simulink model "EngDem"  (R2018a)
settings: configuration reference "cs_ert" (kept outside this file)
settings Model: DataDictionary=EngDem.sldd  Creator=zhoutinglin  LastModifiedBy=zhoutinglin

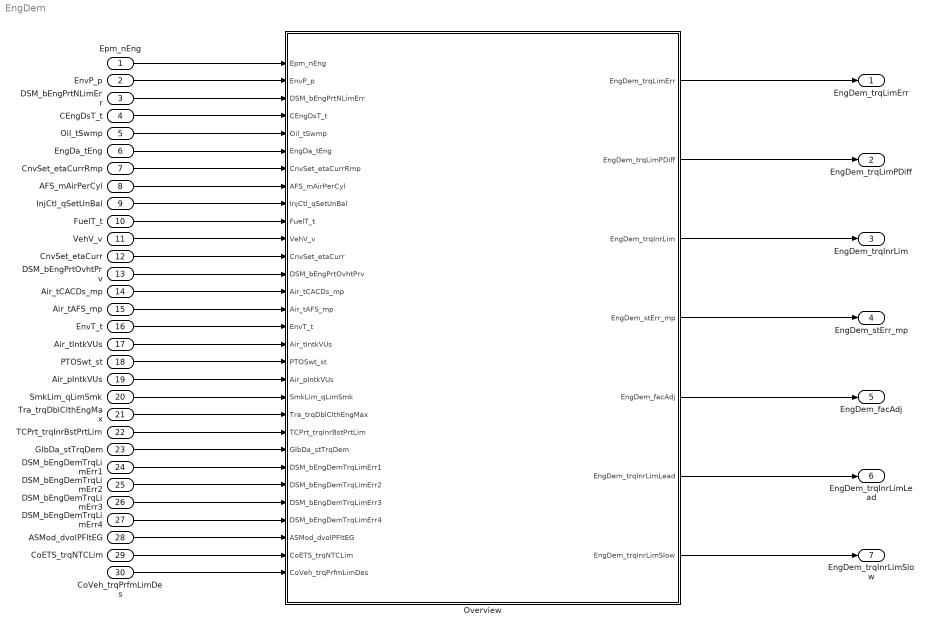
== system EngDem ==
  Epm_nEng : Inport
  EnvP_p : Inport  Port=2
  DSM_bEngPrtNLimErr : Inport  Port=3
  CEngDsT_t : Inport  Port=4
  Oil_tSwmp : Inport  Port=5
  EngDa_tEng : Inport  Port=6
  CnvSet_etaCurrRmp : Inport  Port=7
  AFS_mAirPerCyl : Inport  Port=8
  InjCtl_qSetUnBal : Inport  Port=9
  FuelT_t : Inport  Port=10
  VehV_v : Inport  Port=11
  CnvSet_etaCurr : Inport  Port=12
  DSM_bEngPrtOvhtPrv : Inport  Port=13
  Air_tCACDs_mp : Inport  Port=14
  Air_tAFS_mp : Inport  Port=15
  EnvT_t : Inport  Port=16
  Air_tIntkVUs : Inport  Port=17
  PTOSwt_st : Inport  Port=18
  Air_pIntkVUs : Inport  Port=19
  SmkLim_qLimSmk : Inport  Port=20
  Tra_trqDblClthEngMax : Inport  Port=21
  TCPrt_trqInrBstPrtLim : Inport  Port=22
  GlbDa_stTrqDem : Inport  Port=23
  DSM_bEngDemTrqLimErr1 : Inport  Port=24
  DSM_bEngDemTrqLimErr2 : Inport  Port=25
  DSM_bEngDemTrqLimErr3 : Inport  Port=26
  DSM_bEngDemTrqLimErr4 : Inport  Port=27
  ASMod_dvolPFltEG : Inport  Port=28
  CoETS_trqNTCLim : Inport  Port=29
  CoVeh_trqPrfmLimDes : Inport  Port=30
  Overview : Subsystem
  EngDem_trqLimErr : Outport
  EngDem_trqLimPDiff : Outport  Port=2
  EngDem_trqInrLim : Outport  Port=3
  EngDem_stErr_mp : Outport  Port=4
  EngDem_facAdj : Outport  Port=5
  EngDem_trqInrLimLead : Outport  Port=6
  EngDem_trqInrLimSlow : Outport  Port=7
  wires:
  Epm_nEng/1 -> Overview/1(Epm_nEng)
  EnvP_p/1 -> Overview/2(EnvP_p)
  DSM_bEngPrtNLimErr/1 -> Overview/3(DSM_bEngPrtNLimErr)
  CEngDsT_t/1 -> Overview/4(CEngDsT_t)
  Oil_tSwmp/1 -> Overview/5(Oil_tSwmp)
  EngDa_tEng/1 -> Overview/6(EngDa_tEng)
  CnvSet_etaCurrRmp/1 -> Overview/7(CnvSet_etaCurrRmp)
  AFS_mAirPerCyl/1 -> Overview/8(AFS_mAirPerCyl)
  InjCtl_qSetUnBal/1 -> Overview/9(InjCtl_qSetUnBal)
  FuelT_t/1 -> Overview/10(FuelT_t)
  VehV_v/1 -> Overview/11(VehV_v)
  CnvSet_etaCurr/1 -> Overview/12(CnvSet_etaCurr)
  DSM_bEngPrtOvhtPrv/1 -> Overview/13(DSM_bEngPrtOvhtPrv)
  Air_tCACDs_mp/1 -> Overview/14(Air_tCACDs_mp)
  Air_tAFS_mp/1 -> Overview/15(Air_tAFS_mp)
  EnvT_t/1 -> Overview/16(EnvT_t)
  Air_tIntkVUs/1 -> Overview/17(Air_tIntkVUs)
  PTOSwt_st/1 -> Overview/18(PTOSwt_st)
  Air_pIntkVUs/1 -> Overview/19(Air_pIntkVUs)
  SmkLim_qLimSmk/1 -> Overview/20(SmkLim_qLimSmk)
  Tra_trqDblClthEngMax/1 -> Overview/21(Tra_trqDblClthEngMax)
  TCPrt_trqInrBstPrtLim/1 -> Overview/22(TCPrt_trqInrBstPrtLim)
  GlbDa_stTrqDem/1 -> Overview/23(GlbDa_stTrqDem)
  DSM_bEngDemTrqLimErr1/1 -> Overview/24(DSM_bEngDemTrqLimErr1)
  DSM_bEngDemTrqLimErr2/1 -> Overview/25(DSM_bEngDemTrqLimErr2)
  DSM_bEngDemTrqLimErr3/1 -> Overview/26(DSM_bEngDemTrqLimErr3)
  DSM_bEngDemTrqLimErr4/1 -> Overview/27(DSM_bEngDemTrqLimErr4)
  ASMod_dvolPFltEG/1 -> Overview/28(ASMod_dvolPFltEG)
  CoETS_trqNTCLim/1 -> Overview/29(CoETS_trqNTCLim)
  CoVeh_trqPrfmLimDes/1 -> Overview/30(CoVeh_trqPrfmLimDes)
  Overview/1(EngDem_trqLimErr) -> EngDem_trqLimErr/1
  Overview/2(EngDem_trqLimPDiff) -> EngDem_trqLimPDiff/1
  Overview/3(EngDem_trqInrLim) -> EngDem_trqInrLim/1
  Overview/4(EngDem_stErr_mp) -> EngDem_stErr_mp/1
  Overview/5(EngDem_facAdj) -> EngDem_facAdj/1
  Overview/6(EngDem_trqInrLimLead) -> EngDem_trqInrLimLead/1
  Overview/7(EngDem_trqInrLimSlow) -> EngDem_trqInrLimSlow/1

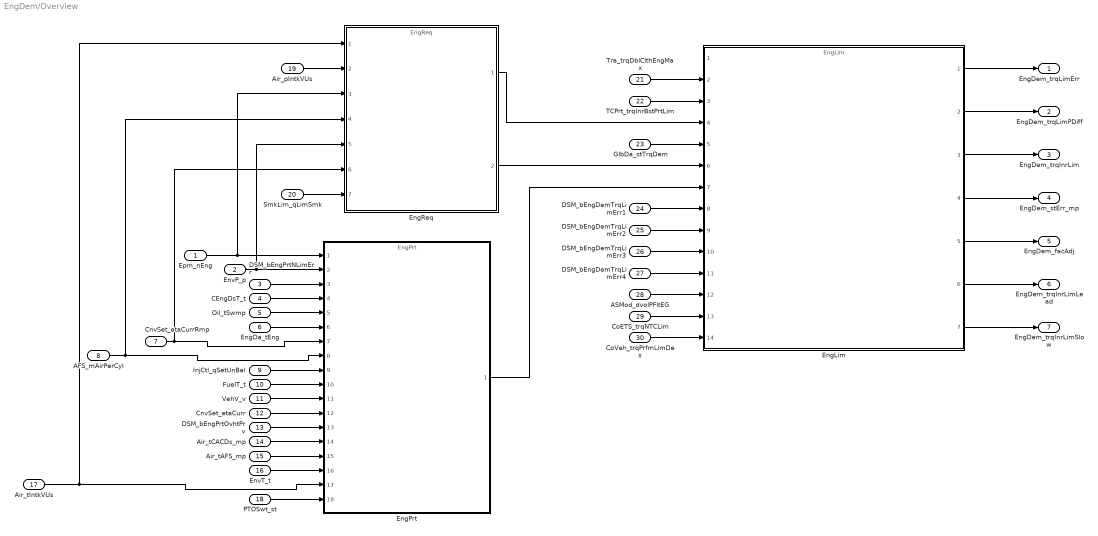
== system EngDem/Overview ==
  Epm_nEng : Inport
  EnvP_p : Inport  Port=2
  DSM_bEngPrtNLimErr : Inport  Port=3
  CEngDsT_t : Inport  Port=4
  Oil_tSwmp : Inport  Port=5
  EngDa_tEng : Inport  Port=6
  CnvSet_etaCurrRmp : Inport  Port=7
  AFS_mAirPerCyl : Inport  Port=8
  InjCtl_qSetUnBal : Inport  Port=9
  FuelT_t : Inport  Port=10
  VehV_v : Inport  Port=11
  CnvSet_etaCurr : Inport  Port=12
  DSM_bEngPrtOvhtPrv : Inport  Port=13
  Air_tCACDs_mp : Inport  Port=14
  Air_tAFS_mp : Inport  Port=15
  EnvT_t : Inport  Port=16
  Air_tIntkVUs : Inport  Port=17
  PTOSwt_st : Inport  Port=18
  Air_pIntkVUs : Inport  Port=19
  SmkLim_qLimSmk : Inport  Port=20
  Tra_trqDblClthEngMax : Inport  Port=21
  TCPrt_trqInrBstPrtLim : Inport  Port=22
  GlbDa_stTrqDem : Inport  Port=23
  DSM_bEngDemTrqLimErr1 : Inport  Port=24
  DSM_bEngDemTrqLimErr2 : Inport  Port=25
  DSM_bEngDemTrqLimErr3 : Inport  Port=26
  DSM_bEngDemTrqLimErr4 : Inport  Port=27
  ASMod_dvolPFltEG : Inport  Port=28
  CoETS_trqNTCLim : Inport  Port=29
  CoVeh_trqPrfmLimDes : Inport  Port=30
  EngLim : ModelReference  ModelNameDialog=EngLim  SimulationMode=Normal  ModelReferenceVersion=1.5
  EngPrt : ModelReference  ModelNameDialog=EngPrt  SimulationMode=Normal  ModelReferenceVersion=1.4
  EngReq : ModelReference  ModelNameDialog=EngReq  SimulationMode=Normal  ModelReferenceVersion=1.5
  EngDem_trqLimErr : Outport
  EngDem_trqLimPDiff : Outport  Port=2
  EngDem_trqInrLim : Outport  Port=3
  EngDem_stErr_mp : Outport  Port=4
  EngDem_facAdj : Outport  Port=5
  EngDem_trqInrLimLead : Outport  Port=6
  EngDem_trqInrLimSlow : Outport  Port=7
  wires:
  EngReq/1 -> EngLim/4
  EngPrt/1 -> EngLim/7
  Epm_nEng/1 -> EngReq/3, EngPrt/1
  EnvP_p/1 -> EngReq/5, EngPrt/2
  DSM_bEngPrtNLimErr/1 -> EngPrt/3
  CEngDsT_t/1 -> EngPrt/4
  Oil_tSwmp/1 -> EngPrt/5
  EngDa_tEng/1 -> EngPrt/6
  CnvSet_etaCurrRmp/1 -> EngReq/6, EngPrt/7
  AFS_mAirPerCyl/1 -> EngReq/4, EngPrt/8
  InjCtl_qSetUnBal/1 -> EngPrt/9
  FuelT_t/1 -> EngPrt/10
  VehV_v/1 -> EngPrt/11
  CnvSet_etaCurr/1 -> EngPrt/12
  DSM_bEngPrtOvhtPrv/1 -> EngPrt/13
  Air_tCACDs_mp/1 -> EngPrt/14
  Air_tAFS_mp/1 -> EngPrt/15
  EnvT_t/1 -> EngPrt/16
  Air_tIntkVUs/1 -> EngReq/1, EngPrt/17
  PTOSwt_st/1 -> EngPrt/18
  Air_pIntkVUs/1 -> EngReq/2
  SmkLim_qLimSmk/1 -> EngReq/7
  Tra_trqDblClthEngMax/1 -> EngLim/2
  TCPrt_trqInrBstPrtLim/1 -> EngLim/3
  GlbDa_stTrqDem/1 -> EngLim/5
  DSM_bEngDemTrqLimErr1/1 -> EngLim/8
  DSM_bEngDemTrqLimErr2/1 -> EngLim/9
  DSM_bEngDemTrqLimErr3/1 -> EngLim/10
  DSM_bEngDemTrqLimErr4/1 -> EngLim/11
  ASMod_dvolPFltEG/1 -> EngLim/12
  CoETS_trqNTCLim/1 -> EngLim/13
  CoVeh_trqPrfmLimDes/1 -> EngLim/14
  EngLim/1 -> EngDem_trqLimErr/1
  EngLim/2 -> EngDem_trqLimPDiff/1
  EngLim/3 -> EngDem_trqInrLim/1
  EngLim/4 -> EngDem_stErr_mp/1
  EngLim/5 -> EngDem_facAdj/1
  EngLim/6 -> EngDem_trqInrLimLead/1
  EngLim/7 -> EngDem_trqInrLimSlow/1
  EngReq/2 -> EngLim/6
